simulink model "Single_Stage_Grid_Connected_Single_Phase_PV_Inverter"  (R2024a)
settings: Solver=FixedStepAuto  StartTime=0.0  StopTime=3.5  FixedStep=1e-6  RelTol=1e-3
libraries: spsIGBTDiodeLib x4, spsSeriesRLCBranchLib x4, spsCurrentMeasurementLib x2, spsFirstOrderFilterLib x2, slpidlib x2, spsVoltageMeasurementLib x2, spsACVoltageSourceLib x1, spsAlphaBetaZerotodq0Lib x1, spsPVArrayLib x1, simulink x1, spsTriangleGeneratorLib x1, sps_lib x1
settings Model: Creator=Vande  LastModifiedBy=Vande

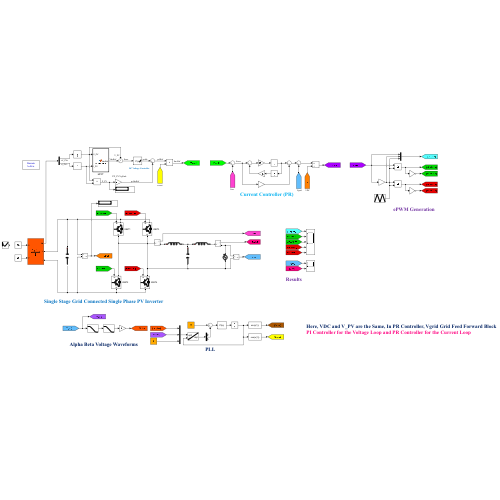
[thumbnail: Simulink's stored preview of the top-level diagram]
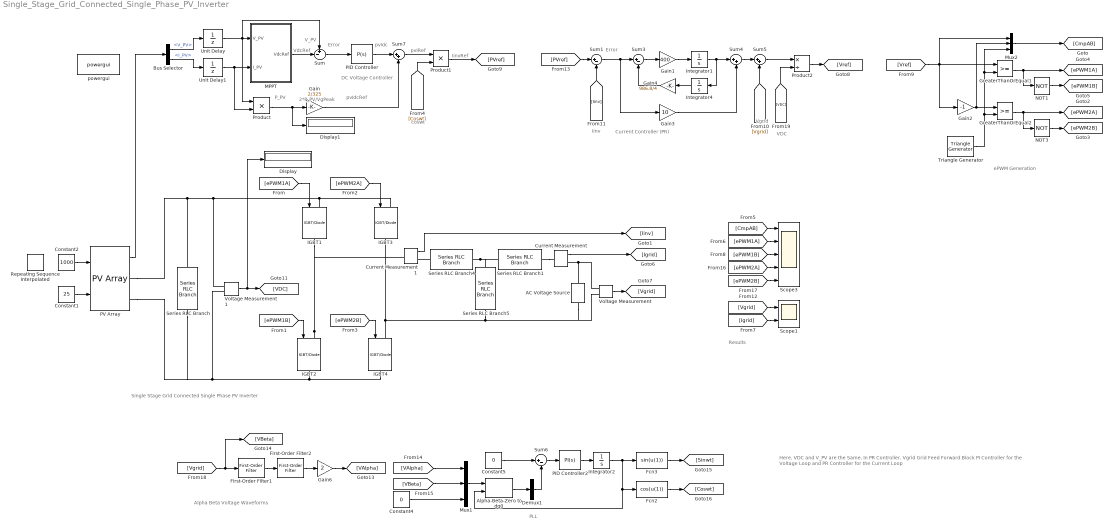
== system Single_Stage_Grid_Connected_Single_Phase_PV_Inverter ==
  note: ePWM Generation
  note: Results
  note: Single Stage Grid Connected Single Phase PV Inverter
  note: PLL
  note: Here, VDC and V_PV are the Same, In PR Controller, Vgrid Grid Feed Forward Block
      | PI Controller for the Voltage Loop and PR Controller for the Current Loop
  note: Alpha Beta Voltage Waveforms
  note: Current Controller (PR)
  note: V_PV
  note: Error
  note: DC Voltage Controller
  note: P_PV
  note: pvIdcRef
  note: pvIdc
  note: pvIRef
  note: IinvRef
  note: Error
  note: coswt
  note: Iinv
  note: Vgrid
  note: VDC
  note: 2*P_PV/VgPeak
  note: VdcRef
  AC Voltage Source : spsACVoltageSourceLib/AC Voltage Source  Amplitude=325  Phase=0  Frequency=50  SampleTime=0  Measurements=None  BusType=swing  Pref=10e3  Qref=0  Qmin=-inf  Qmax=+inf
  Alpha-Beta-Zero to dq0 : spsAlphaBetaZerotodq0Lib/Alpha-Beta-Zero to dq0  Alignment=90 degrees behind phase A axis
  Bus Selector : BusSelector  OutputSignals=V_PV,I_PV
  Constant1 : Constant  Value=25
  Constant2 : Constant  Value=1000
  Constant4 : Constant  Value=0
  Constant5 : Constant  Value=0
  Current Measurement : spsCurrentMeasurementLib/Current Measurement  PhasorSimulation=off  OutputType=Complex  PSBequivalent=0
  Current Measurement1 : spsCurrentMeasurementLib/Current Measurement  PhasorSimulation=off  OutputType=Complex  PSBequivalent=0
  Demux1 : Demux  Outputs=3
  Display : Display
  Display1 : Display
  Fcn2 : Fcn  Expr=cos(u(1))
  Fcn3 : Fcn  Expr=sin(u(1))
  First-Order Filter1 : spsFirstOrderFilterLib/First-Order Filter  FilterType=Lowpass  Tc=1/(2*pi*50)  Ts=0  Initialize=off  Vac_Init=[0, 0, 60]  Vdc_Init=0  PlotResponse=off  FreqRange="[0,  200,  1]"
  First-Order Filter2 : spsFirstOrderFilterLib/First-Order Filter  FilterType=Lowpass  Tc=1/(2*pi*50)  Ts=0  Initialize=off  Vac_Init=[0, 0, 60]  Vdc_Init=0  PlotResponse=off  FreqRange="[0,  200,  1]"
  Gain : Gain  Gain=2/325
  Gain1 : Gain  Gain=400
  Gain2 : Gain  Gain=-1
  Gain3 : Gain  Gain=10
  Gain4 : Gain  Gain=986.8/4
  Gain6 : Gain  Gain=2
  GreaterThanOrEqual1 : RelationalOperator  OutDataTypeStr=boolean  RndMeth=Simplest  InputSameDT=off
  GreaterThanOrEqual2 : RelationalOperator  OutDataTypeStr=boolean  RndMeth=Simplest  InputSameDT=off
  IGBT{1..4} (4 alike) : spsIGBTDiodeLib/IGBT//Diode  Ron=1e-3  Rs=1e5  Cs=inf  Measurements=off
  Integrator1 : Integrator
  Integrator2 : Integrator
  Integrator4 : Integrator
  MPPT : MATLAB Function  TreatAsAtomicUnit=on
  Mux1 : Mux  Inputs=3
  Mux2 : Mux  Inputs=3
  NOT1 : Logic  Operator=NOT  IconShape=distinctive  AllPortsSameDT=off  OutDataTypeStr=boolean
  NOT3 : Logic  Operator=NOT  IconShape=distinctive  AllPortsSameDT=off  OutDataTypeStr=boolean
  PID Controller : slpidlib/PID Controller  Controller=P  Form=Parallel  TimeDomain=Continuous-time  UseExternalTs=off  SampleTime=-1  IntegratorMethod=Forward Euler  FilterMethod=Forward Euler  ControllerParametersSource=internal  P=0.075  I=0.075  UseKiTs=off  D=0  UseExternalDerivativeSource=off  N=100  UseFilter=on  TunerSelectOption=Transfer Function Based (PID Tuner App)  InitialConditionSource=internal  InitialConditionForIntegrator=0  InitialConditionForFilter=0  DifferentiatorICPrevScaledInput=0  ExternalReset=none  TrackingMode=off  Kt=1  LimitOutput=on  SatLimitsSource=internal  UpperSaturationLimit=0.95  LowerSaturationLimit=0  LinearizeAsGain=on  AntiWindupMode=none  Kb=1  LimitIntegrator=off  UpperIntegratorSaturationLimit=inf  LowerIntegratorSaturationLimit=-inf  POutMin=[]  POutMax=[]  IOutMin=[]  IOutMax=[]  DOutMin=[]  DOutMax=[]  NOutMin=[]  NOutMax=[]  SumOutMin=[]  SumOutMax=[]  SaturationOutMin=[]  SaturationOutMax=[]  PParamMin=[]  PParamMax=[]  IParamMin=[]  IParamMax=[]  DParamMin=[]  DParamMax=[]  NParamMin=[]  NParamMax=[]  KbParamMin=[]  KbParamMax=[]  KtParamMin=[]  KtParamMax=[]  KbOutMin=[]  KbOutMax=[]  KtOutMin=[]  KtOutMax=[]  IntegratorOutMin=[]  IntegratorOutMax=[]  FilterOutMin=[]  FilterOutMax=[]  SumI1OutMin=[]  SumI1OutMax=[]  SumI2OutMin=[]  SumI2OutMax=[]  SumI3OutMin=[]  SumI3OutMax=[]  SumI4OutMin=[]  SumI4OutMax=[]  SumDOutMin=[]  SumDOutMax=[]  DifferentiatorOutMin=[]  DifferentiatorOutMax=[]  FilterDiffOutCoefMin=[]  FilterDiffOutCoefMax=[]  ReciprocalOutMin=[]  ReciprocalOutMax=[]  SumDenOutMin=[]  SumDenOutMax=[]  SumNumOutMin=[]  SumNumOutMax=[]  DivideOutMin=[]  DivideOutMax=[]  UdiffTsProdOutMin=[]  UdiffTsProdOutMax=[]  NTsProdOutMin=[]  NTsProdOutMax=[]  UintegralTsProdOutMin=[]  UintegralTsProdOutMax=[]  UngainTsProdOutMin=[]  UngainTsProdOutMax=[]  ClampingZeroOutDataTypeStr=Inherit: Inherit via back propagation  ClampingZeroOutMin=[]  ClampingZeroOutMax=[]  FilterDenConstantOutDataTypeStr=Inherit: Inherit via back propagation  FilterDenConstantOutMin=[]  FilterDenConstantOutMax=[]  PCopyOutDataTypeStr=Inherit: Inherit via back propagation  PCopyOutMin=[]  PCopyOutMax=[]  NCopyOutDataTypeStr=Inherit: Inherit via back propagation  NCopyOutMin=[]  NCopyOutMax=[]  IntegratorContinuousStateAttributes=''  IntegratorStateMustResolveToSignalObject=off  IntegratorRTWStateStorageClass=Auto  FilterContinuousStateAttributes=''  FilterStateMustResolveToSignalObject=off  FilterRTWStateStorageClass=Auto  ParallelPVariant=InternalParameters  IdealPVariant=Disabled  IVariant=Disabled  DVariant=Disabled  IntegratorVariant=Disabled  SatVariant=Enabled  AWVariant=Disabled  PCopyVariant=Disabled  TRVariant=Disabled  FdbkBlocksVariant=Forward  IdealPFdbkVariant=Disabled  SatFdbkVariant=Disabled  DerivativeFilterVariant=Disabled  NVariant=Disabled  NCopyVariant=Disabled_SignalSpec  FilterICVariant=Disabled  IntegratorICVariant=Disabled  ExternalResetVariant=Disabled  TRSumVariant=Passthrough  SumFdbkVariant=Disabled  SumVariant=Passthrough_P  TsampFilterVariant=InternalTs  TsampNgainVariant=Passthrough  TsampIntegralVariant=Disabled_SignalSpec  ExternalSaturationOutDataTypeStr=Inherit: Same as second input  DerivativeSourceVariant=Disabled
  PID Controller2 : slpidlib/PID Controller  Controller=PI  Form=Parallel  TimeDomain=Continuous-time  UseExternalTs=off  SampleTime=-1  IntegratorMethod=Forward Euler  FilterMethod=Forward Euler  ControllerParametersSource=internal  P=10  I=5000  UseKiTs=off  D=0  UseExternalDerivativeSource=off  N=100  UseFilter=on  TunerSelectOption=Transfer Function Based (PID Tuner App)  InitialConditionSource=internal  InitialConditionForIntegrator=0  InitialConditionForFilter=0  DifferentiatorICPrevScaledInput=0  ExternalReset=none  TrackingMode=off  Kt=1  LimitOutput=off  SatLimitsSource=internal  UpperSaturationLimit=inf  LowerSaturationLimit=-inf  LinearizeAsGain=on  AntiWindupMode=none  Kb=1  LimitIntegrator=off  UpperIntegratorSaturationLimit=inf  LowerIntegratorSaturationLimit=-inf  POutMin=[]  POutMax=[]  IOutMin=[]  IOutMax=[]  DOutMin=[]  DOutMax=[]  NOutMin=[]  NOutMax=[]  SumOutMin=[]  SumOutMax=[]  SaturationOutMin=[]  SaturationOutMax=[]  PParamMin=[]  PParamMax=[]  IParamMin=[]  IParamMax=[]  DParamMin=[]  DParamMax=[]  NParamMin=[]  NParamMax=[]  KbParamMin=[]  KbParamMax=[]  KtParamMin=[]  KtParamMax=[]  KbOutMin=[]  KbOutMax=[]  KtOutMin=[]  KtOutMax=[]  IntegratorOutMin=[]  IntegratorOutMax=[]  FilterOutMin=[]  FilterOutMax=[]  SumI1OutMin=[]  SumI1OutMax=[]  SumI2OutMin=[]  SumI2OutMax=[]  SumI3OutMin=[]  SumI3OutMax=[]  SumI4OutMin=[]  SumI4OutMax=[]  SumDOutMin=[]  SumDOutMax=[]  DifferentiatorOutMin=[]  DifferentiatorOutMax=[]  FilterDiffOutCoefMin=[]  FilterDiffOutCoefMax=[]  ReciprocalOutMin=[]  ReciprocalOutMax=[]  SumDenOutMin=[]  SumDenOutMax=[]  SumNumOutMin=[]  SumNumOutMax=[]  DivideOutMin=[]  DivideOutMax=[]  UdiffTsProdOutMin=[]  UdiffTsProdOutMax=[]  NTsProdOutMin=[]  NTsProdOutMax=[]  UintegralTsProdOutMin=[]  UintegralTsProdOutMax=[]  UngainTsProdOutMin=[]  UngainTsProdOutMax=[]  ClampingZeroOutDataTypeStr=Inherit: Inherit via back propagation  ClampingZeroOutMin=[]  ClampingZeroOutMax=[]  FilterDenConstantOutDataTypeStr=Inherit: Inherit via back propagation  FilterDenConstantOutMin=[]  FilterDenConstantOutMax=[]  PCopyOutDataTypeStr=Inherit: Inherit via back propagation  PCopyOutMin=[]  PCopyOutMax=[]  NCopyOutDataTypeStr=Inherit: Inherit via back propagation  NCopyOutMin=[]  NCopyOutMax=[]  IntegratorContinuousStateAttributes=''  IntegratorStateMustResolveToSignalObject=off  IntegratorRTWStateStorageClass=Auto  FilterContinuousStateAttributes=''  FilterStateMustResolveToSignalObject=off  FilterRTWStateStorageClass=Auto  ParallelPVariant=InternalParameters  IdealPVariant=Disabled  IVariant=InternalParameters  DVariant=Disabled  IntegratorVariant=Continuous  SatVariant=Disabled  AWVariant=Passthrough  PCopyVariant=Disabled  TRVariant=Disabled  FdbkBlocksVariant=Forward  IdealPFdbkVariant=Disabled  SatFdbkVariant=Disabled  DerivativeFilterVariant=Disabled  NVariant=Disabled  NCopyVariant=Disabled_SignalSpec  FilterICVariant=Disabled  IntegratorICVariant=InternalICs  ExternalResetVariant=Disabled  TRSumVariant=Passthrough  SumFdbkVariant=Disabled  SumVariant=Sum_PI  TsampFilterVariant=InternalTs  TsampNgainVariant=Passthrough  TsampIntegralVariant=Disabled_SignalSpec  ExternalSaturationOutDataTypeStr=Inherit: Same as second input  DerivativeSourceVariant=Disabled
  PV Array : spsPVArrayLib/PV Array  Npar=1  Nser=11  PlotType=array @ 25 deg.C & specified irradiances  S_vec="[ 1000  500  100 ]"  Temp_C_vec="[ 45 25  ]"  ModuleName=Zytech Engineering Technology ZT190S  PlotWhenSelected=off  Pm=190.1592  Ncell=72  Voc=44.86  Isc=5.5  Vm=37.73  Im=5.04  beta_Voc_pc=-0.364  alpha_Isc_pc=0.102  beta_Voc=-0.16329  alpha_Isc=0.00561  IL=5.5086  I0=2.2516e-10  nI=1.0158  Rsh=179.2693  Rs=0.2794  RobustModel=off  RobustCellTemperature=313.3991  BAL=on  Tc=1e-6  Tfilter=1e-6
  Product : Product
  Product1 : Product
  Product2 : Product  Inputs=*/
  Repeating Sequence Interpolated : simulink/Sources/Repeating Sequence Interpolated  OutValues=[1000 500 300 1000].'  TimeValues=[0 0.5 1.5 3.5].'  LookUpMeth=Interpolation-Use End Values  tsamp=0.01  OutMin=[]  OutMax=[]  OutDataTypeStr=double  OutputDataTypeScalingMode=double  OutDataType=fixdt(0,8)  OutScaling=2^-10
  Scope1 : Scope  NumInputPorts=2
  Scope3 : Scope  NumInputPorts=5
  Series RLC Branch : spsSeriesRLCBranchLib/Series RLC Branch  LConnTagsString=__new0  RConnTagsString=__new0  BranchType=C  Resistance=1  Inductance=1e-3  SetiL0=off  InitialCurrent=0  Capacitance=600e-6  Setx0=on  InitialVoltage=493.5  Measurements=None
  Series RLC Branch1 : spsSeriesRLCBranchLib/Series RLC Branch  LConnTagsString=__new0  RConnTagsString=__new0  BranchType=L  Resistance=2  Inductance=6.39e-3  SetiL0=off  InitialCurrent=0  Capacitance=1e-6  Setx0=off  InitialVoltage=0  Measurements=None
  Series RLC Branch4 : spsSeriesRLCBranchLib/Series RLC Branch  LConnTagsString=__new0  RConnTagsString=__new0  BranchType=L  Resistance=2  Inductance=2.03e-3  SetiL0=off  InitialCurrent=0  Capacitance=1e-6  Setx0=off  InitialVoltage=0  Measurements=None
  Series RLC Branch5 : spsSeriesRLCBranchLib/Series RLC Branch  LConnTagsString=__new0  RConnTagsString=__new0  BranchType=C  Resistance=1  Inductance=1e-3  SetiL0=off  InitialCurrent=0  Capacitance=6.02e-6  Setx0=off  InitialVoltage=0  Measurements=None
  Sum : Sum  Inputs=+-|
  Sum1 : Sum  Inputs=|+-
  Sum3 : Sum  Inputs=|+-
  Sum4 : Sum  Inputs=|++
  Sum5 : Sum  Inputs=|++
  Sum6 : Sum  Inputs=|+-
  Sum7 : Sum  Inputs=|++
  Triangle Generator : spsTriangleGeneratorLib/Triangle Generator  Freq=10000  Phase=0  Ts=0
  Unit Delay : UnitDelay  SampleTime=1e-4  HasFrameUpgradeWarning=on
  Unit Delay1 : UnitDelay  SampleTime=1e-4  HasFrameUpgradeWarning=on
  Voltage Measurement : spsVoltageMeasurementLib/Voltage Measurement  PhasorSimulation=off  OutputType=Complex  PSBequivalent=0
  Voltage Measurement1 : spsVoltageMeasurementLib/Voltage Measurement  PhasorSimulation=off  OutputType=Complex  PSBequivalent=0
  powergui : sps_lib/powergui  Priority=1  SimulationMode=Discrete  SampleTime=1e-6  frequency=60  Iterations=50  frequencyindice=0  Pbase=100e6  ErrMax=1e-4  UnitsV=kV  UnitsW=MW  buscounter=0  FunctionMessages=off  echomessages=off  EnableUseOfTLC=off  CurrentSourceSwitches=off  DisableSnubberDevices=off  DisableRonSwitches=off  DisableVfSwitches=off  DisplayEquations=off  AutomaticDiscreteSolvers=off  SolverType=Tustin/Backward Euler (TBE)  Interpol=off  ExternalGateDelay=off  methode=off  Ts=100  x0status=blocks  SPID=on  SwTol=0  HookPort=off  NonlinearTolerance=1e-4  nMaxIteration=100  ContinueOnMaxIteration=off  RestoreLinks=warning  ResistiveCurrentMeasurement=off  Frange=[0:2:500]  Ylog=off  Xlog=on  ShowGrid=off  save=off  variable=ZData  structure=0  ZoomFFT=off  StartTime=0.0  cycles=1  DisplayStyle=1  fundamental=60  FreqAxis=off  MaxFrequency=1000  frequencyindicesteady=1  RmsSteady=1  display=off
  wires:
  Sum5/1 -> Product2/1
  [PVref] -> Sum1/1
  NOT3/1 -> [ePWM2B]
  Gain4/1 -> Sum3/2
  Sum1/1 -> Sum3/1, Gain3/1
  Gain3/1 -> Sum4/2
  Sum4/1 -> Sum5/1
  Integrator4/1 -> Gain4/1
  Mux2/1 -> [CmpAB]
  GreaterThanOrEqual2/1 -> [ePWM2A], NOT3/1
  Gain1/1 -> Integrator1/1
  Product2/1 -> [Vref]
  [Vgrid] -> Sum5/2
  GreaterThanOrEqual1/1 -> [ePWM1A], NOT1/1
  Triangle Generator/1 -> GreaterThanOrEqual2/2, GreaterThanOrEqual1/2, Mux2/3
  Voltage Measurement/1 -> [Vgrid]
  [Iinv] -> Sum1/2
  [CmpAB] -> Scope3/1
  [Vref] -> Gain2/1, Mux2/1, GreaterThanOrEqual1/1
  [ePWM2B] -> IGBT4/1
  Current Measurement/1 -> [Igrid]
  Current Measurement1/1 -> [Iinv]
  [ePWM1A] -> Scope3/2
  Unit Delay1/1 -> Product/2, MPPT/2(I_PV)
  Bus Selector/1 -> Unit Delay/1  "<V_PV>"
  Sum/1 -> PID Controller/1
  Voltage Measurement1/1 -> [VDC], Display/1
  Bus Selector/2 -> Unit Delay1/1  "<I_PV>"
  Product/1 -> Gain/1, Display1/1
  MPPT/1(VdcRef) -> Sum/2
  [Vgrid] -> Scope1/1
  [ePWM2A] -> Scope3/4
  NOT1/1 -> [ePWM1B]
  PID Controller/1 -> Sum7/1
  Gain2/1 -> GreaterThanOrEqual2/1, Mux2/2
  [ePWM1B] -> Scope3/3
  [ePWM1A] -> IGBT1/1
  [ePWM2B] -> Scope3/5
  [Igrid] -> Scope1/2
  [ePWM2A] -> IGBT3/1
  [ePWM1B] -> IGBT2/1
  PV Array/1 -> Bus Selector/1
  Integrator1/1 -> Sum4/1, Integrator4/1
  Constant1/1 -> PV Array/2
  Unit Delay/1 -> Product/1, Sum/1, MPPT/1(V_PV)
  First-Order Filter1/1 -> First-Order Filter2/1
  PID Controller2/1 -> Integrator2/1
  Sum6/1 -> PID Controller2/1
  Constant5/1 -> Sum6/1
  Fcn2/1 -> [Coswt]
  Gain6/1 -> [VAlpha]
  Demux1/2 -> Sum6/2
  Integrator2/1 -> Fcn3/1, Fcn2/1, Alpha-Beta-Zero to dq0/2
  Constant4/1 -> Mux1/3
  [VBeta] -> Mux1/2
  [VAlpha] -> Mux1/1
  [Vgrid] -> First-Order Filter1/1, [VBeta]
  Alpha-Beta-Zero to dq0/1 -> Demux1/1
  Fcn3/1 -> [Sinwt]
  First-Order Filter2/1 -> Gain6/1
  Mux1/1 -> Alpha-Beta-Zero to dq0/1
  Sum7/1 -> Product1/1
  Product1/1 -> [PVref]
  Sum3/1 -> Gain1/1
  [VDC] -> Product2/2
  Gain/1 -> Sum7/2
  Constant2/1 -> PV Array/1
  [Coswt] -> Product1/2
  connections:
  IGBT4/LConn1 -- Voltage Measurement/LConn2 -- AC Voltage Source/LConn1 -- Series RLC Branch5/RConn1 -- IGBT3/RConn1
  IGBT2/LConn1 -- IGBT1/RConn1 -- Current Measurement1/LConn1
  IGBT4/RConn1 -- Series RLC Branch/RConn1 -- PV Array/RConn2 -- Voltage Measurement1/LConn2 -- IGBT2/RConn1
  Voltage Measurement/LConn1 -- AC Voltage Source/RConn1 -- Current Measurement/RConn1
  PV Array/RConn1 -- Series RLC Branch/LConn1 -- Voltage Measurement1/LConn1 -- IGBT1/LConn1 -- IGBT3/LConn1
  Series RLC Branch4/RConn1 -- Series RLC Branch1/LConn1 -- Series RLC Branch5/LConn1
  Series RLC Branch1/RConn1 -- Current Measurement/LConn1
  Series RLC Branch4/LConn1 -- Current Measurement1/RConn1

== matlab function Single_Stage_Grid_Connected_Single_Phase_PV_Inverter/MPPT ==
  data: V_PV input; VdcRef output; I_PV input
% Perturb and Observe MPPT Algorithm
function VdcRef = VdcRefGen(V_PV, I_PV) % VdcRef is the Reference Voltage V or MPPT Output, I are the MPPT Inputs

% Define Constants
VdcRefMax = 493.5;       % Maximum Reference Voltage (493.5 Open Circuit Voltage (Voc) for 1000 Irradiances of PV Array)
VdcRefMin = 0;           % Minimum Reference Voltage
VdcRefInit = 415;        % Initial Reference Voltage (415 MPP for 1000 Irradiances)
deltaVdcRef = 1;         % Step Size for Reference Voltage Adjustment

% Declare Persistent Variables to Store Previous Values
persistent Vprev Pprev VdcRefprev;

% Specify Data Type for Consistency (Not Used Directly in This Code)
dataType = 'double';

% Initialize Persistent Variables If They Are Empty (First Function Call)
if isempty(Vprev)
    V_PVprev = 0;                % Previous Voltage
    P_PVprev = 0;                % Previous Power
    VdcRefprev = VdcRefInit;     % Previous Reference Voltage
end

% Calculate Current Power and its Difference From the Previous Power
P_PV = V_PV * I_PV;          % Current Power
dV = V_PV - V_PVprev;        % Change in Voltage
dP = P_PV - P_PVprev;        % Change in Power

% Perturb and Observe Algorithm to Adjust VdcRef
if dP ~= 0
    % Check If There is Change in Power
    if dP < 0
        % If Power Has Decreased
        if dV < 0
            % If Voltage Has Decreased, Increase Reference Voltage
            VdcRef = VdcRefprev + deltaVdcRef; % Increase Reference Voltage
        else
            % If Voltage Has Increased, Decrease Reference Voltage
            VdcRef = VdcRefprev - deltaVdcRef; % Decrease Reference Voltage
        end
    else
        % If Power Has Increased
        if dV < 0
            % If Voltage Has Decreased, Decrease Reference Voltage
            VdcRef = VdcRefprev - deltaVdcRef; % Decrease Reference Voltage
        else
            % If Voltage Has Increased, Increase Reference Voltage
            VdcRef = VdcRefprev + deltaVdcRef; % Increase Reference Voltage
        end
    end
else
    % If There is No Change in Power, Keep Reference Voltage Unchanged
    VdcRef = VdcRefprev; % No Change in Power, Keep Reference Voltage Unchanged
end

% Ensure VdcRef Stays within the Defined Limits
if VdcRef >= VdcRefMax || VdcRef <= VdcRefMin
    % If the Teference Voltage Exceeds Limits, Revert to Previous Reference Voltage
    VdcRef = VdcRefprev; % Revert to Previous Reference Voltage if Limits are Exceeded
end

% Update Persistent Variables for the Next Iteration
VdcRefprev = VdcRef;     % Store Current Reference Voltage
V_PVprev = V_PV;            % Store Current Voltage
P_PVprev = P_PV;            % Store Current Power
